simulink model "tanque_sim"  (R2017a)
settings: Solver=VariableStepAuto  StartTime=0.0  StopTime=10.0  RelTol=1e-3
settings Model: Creator=Martin  LastModifiedBy=Alan

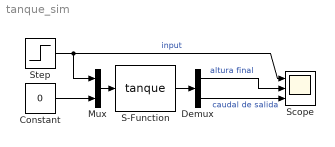
== system tanque_sim ==
  Constant : Constant  Value=0
  Demux : Demux  Outputs=2
  Mux : Mux  Inputs=2
  S-Function : S-Function  FunctionName=tanque  Parameters=0.5,10,3,1  SFunctionDeploymentMode=off  EnableBusSupport=off
  Scope : Scope  NumInputPorts=3
  Step : Step  SampleTime=0
  wires:
  Mux/1 -> S-Function/1
  Constant/1 -> Mux/2
  S-Function/1 -> Demux/1
  Demux/1 -> Scope/2  "altura final"
  Demux/2 -> Scope/3  "caudal de salida"
  Step/1 -> Scope/1, Mux/1  "input"
